simulink model "sfunHeatExchangerExample"  (Simulink 7.6)
settings: Solver=VariableStepDiscrete  StartTime=0.0  StopTime=3600  MaxStep=60  RelTol=1e-3
undefined symbols (not defined in the file): ua0, uam, uat
libraries: carnot x2
settings Model: Creator=drhf  LastModifiedBy=drhf

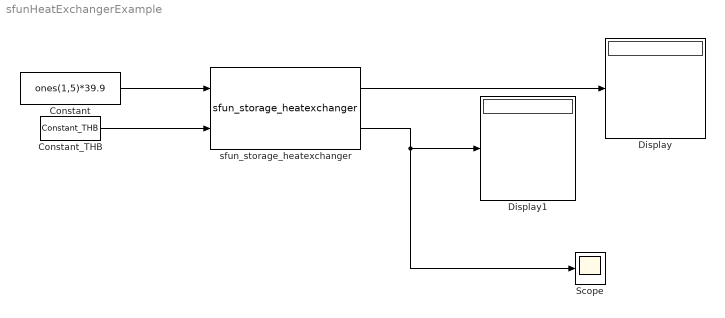
== system sfunHeatExchangerExample ==
  Constant : Constant  Value=ones(1,5)*39.9
  Constant_THB : carnot/Source/Simple/Constant_THB  SystemSampleTime=-1  t=40  mdot=1/3600  p=1e5  mID=No Pressure Drop  fluid=water  mix=0  dia=0.02  hgt=0
  Display : Display
  Display1 : Display
  Scope : Scope
  sfun_storage_heatexchanger : carnot/Basic/Thermal_Models/sfun_storage_heatexchanger  SystemSampleTime=-1  idn=heat transfer from data fit  nodes=5  inlet=1  outlet=5  pp=[100, 0, 0, 0,0,0,0] % [ua0, uam, uat, 0,0,0,0]
  wires:
  Constant/1 -> sfun_storage_heatexchanger/1
  Constant_THB/1 -> sfun_storage_heatexchanger/2
  sfun_storage_heatexchanger/1 -> Display/1
  sfun_storage_heatexchanger/2 -> Display1/1, Scope/1
